simulink model "Q2_b1"  (R2016b)
settings: Solver=ode45  StartTime=0.0  StopTime=0.4  RelTol=1e-10  AbsTol=1e-10  EnableMultiTasking=on
libraries: cstblocks x3
settings Model: Creator=yarde_000  LastModifiedBy=nadav
settings DataIOCC: LimitDataPoints=on  SaveFormat=Array
settings OptimizationCC: LifeSpan=inf
settings DebuggingCC: SFUnexpectedBacktrackingDiag=warning  SFNoUnconditionalDefaultTransitionDiag=warning  SFExecutionAtInitializationDiag=none
settings HardwareCC: ProdBitPerPointer=32  ProdBitPerSizeT=32  ProdBitPerPtrDiffT=32  ProdLargestAtomicFloat=None  ProdIntDivRoundTo=Undefined  ProdEndianess=Unspecified  ProdWordSize=32  ProdHWDeviceType=32-bit Generic
settings ModelReferenceCC: PropagateSignalLabelsOutOfModel=off
settings GRTTargetCC: TargetLangStandard=C89/C90 (ANSI)  GeneratePreprocessorConditionals=Disable all
settings ConfigComp: CovMetricSettings=dw  CovHtmlReporting=on  CovSaveCumulativeToWorkspaceVar=on  CovSaveSingleToWorkspaceVar=on  CovExternalEMLEnable=off

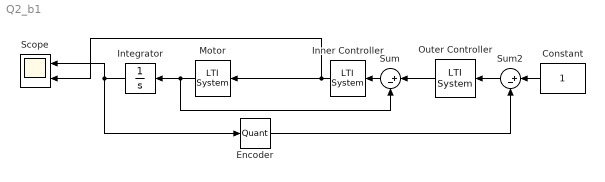
== system Q2_b1 ==
  Constant : Constant
  Encoder : Quantizer  QuantizationInterval=enc_res
  Inner Controller : cstblocks/LTI System  sys=Cpi  IC=[]
  Integrator : Integrator
  Motor : cstblocks/LTI System  sys=P  IC=[]
  Outer Controller : cstblocks/LTI System  sys=Cp  IC=[]
  Scope : Scope  NumInputPorts=2
  Sum : Sum  Inputs=|+-
  Sum2 : Sum  Inputs=|+-
  wires:
  Sum/1 -> Inner Controller/1
  Outer Controller/1 -> Sum/1
  Inner Controller/1 -> Motor/1, Scope/2
  Motor/1 -> Integrator/1, Sum/2
  Integrator/1 -> Encoder/1, Scope/1
  Sum2/1 -> Outer Controller/1
  Constant/1 -> Sum2/1
  Encoder/1 -> Sum2/2
